simulink model "two_wheel_model_control"  (R2020a)
settings: Solver=VariableStepAuto  StartTime=0.0  StopTime=10.0  RelTol=1e-3
values from neighbouring files (symbols this model uses):
  A23 = -b*d/(a*c-b*e)    (= -1.9886253421)    [two_wheel_model.m]
  A43 = a*d/(a*c-b*e)    (= 33.2052798573)    [two_wheel_model.m]
  B21 = (c+b)/(a*c-b*e)    (= 1.96075852141)    [two_wheel_model.m]
  B22 = (c+b)/(a*c-b*e)    (= 1.96075852141)    [two_wheel_model.m]
  B41 = -(e+a)/(a*c-b*e)    (= -10.2174481788)    [two_wheel_model.m]
  B42 = -(e+a)/(a*c-b*e)    (= -10.2174481788)    [two_wheel_model.m]
  B61 = f    (= 7.73512853901)    [two_wheel_model.m]
  B62 = -f    (= -7.73512853901)    [two_wheel_model.m]
  K = lqr(A,B,Q,R)    [two_wheel_model.m]
  V = 1.5    [two_wheel_model.m]
  Yaw = 0.523    [two_wheel_model.m]
settings Model: Creator=solitude  LastModifiedBy=solitude

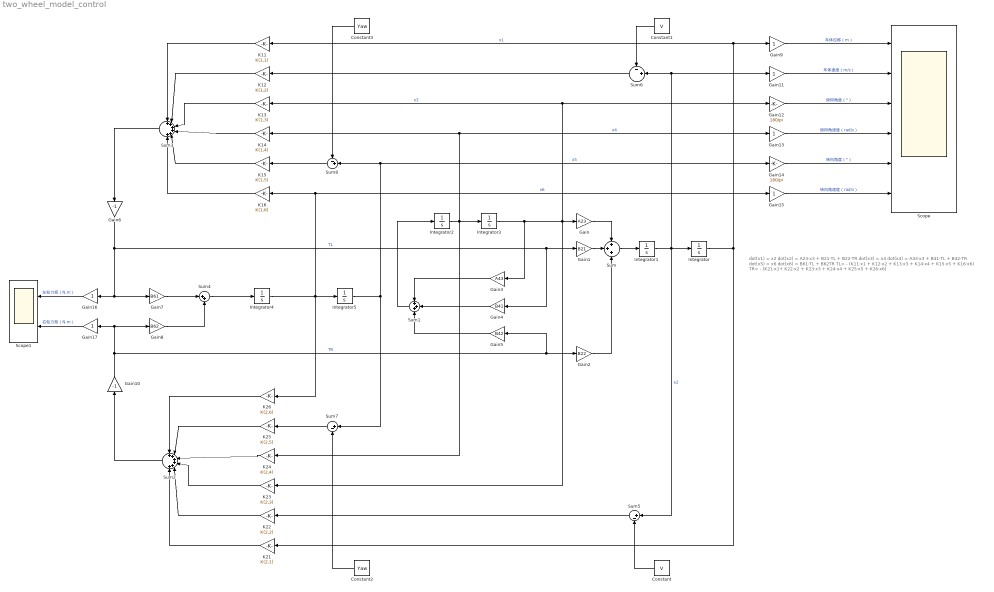
== system two_wheel_model_control ==
  note: dot(x1) = x2
      |
      | dot(x2) = A23·x3 + B21·TL + B22·TR
      |
      | dot(x3) = x4
      |
      | dot(x4) = A43·x3 + B41·TL + B42·TR
      |
      | dot(x5) = x6
      |
      | dot(x6) = B61·TL + B62TR
      |
      | TL= - (K11·x1 + K12·x2 + K13·x3 + K14·x4 + K15·x5 + K16·x6)
      |
      | TR= - (K21·x1+ K22·x2 + K23·x3 + K24·x4 + K25·x5 + K26·x6)
  Constant : Constant  Value=V
  Constant1 : Constant  Value=V
  Constant2 : Constant  Value=Yaw
  Constant3 : Constant  Value=Yaw
  Gain : Gain  Gain=A23
  Gain1 : Gain  Gain=B21
  Gain10 : Gain  Gain=-1
  Gain{9,11,13,15..17} (6 alike) : Gain
  Gain12 : Gain  Gain=180/pi
  Gain14 : Gain  Gain=180/pi
  Gain2 : Gain  Gain=B22
  Gain3 : Gain  Gain=A43
  Gain4 : Gain  Gain=B41
  Gain5 : Gain  Gain=B42
  Gain6 : Gain  Gain=-1
  Gain7 : Gain  Gain=B61
  Gain8 : Gain  Gain=B62
  Integrator{,1..5} (6 alike) : Integrator
  K11 : Gain  Gain=K(1,1)
  K12 : Gain  Gain=K(1,2)
  K13 : Gain  Gain=K(1,3)
  K14 : Gain  Gain=K(1,4)
  K15 : Gain  Gain=K(1,5)
  K16 : Gain  Gain=K(1,6)
  K21 : Gain  Gain=K(2,1)
  K22 : Gain  Gain=K(2,2)
  K23 : Gain  Gain=K(2,3)
  K24 : Gain  Gain=K(2,4)
  K25 : Gain  Gain=K(2,5)
  K26 : Gain  Gain=K(2,6)
  Scope : Scope  NumInputPorts=6
  Scope1 : Scope  NumInputPorts=2
  Sum : Sum  Inputs=+++
  Sum1 : Sum  Inputs=+++
  Sum2 : Sum  Inputs=++++++
  Sum3 : Sum  Inputs=++++++
  Sum4 : Sum  Inputs=|++
  Sum5 : Sum  Inputs=|+-
  Sum6 : Sum  Inputs=-+|
  Sum7 : Sum  Inputs=|+-
  Sum8 : Sum  Inputs=-+|
  wires:
  Integrator/1 -> K11/1, Gain9/1, K21/1  "x1"
  Integrator1/1 -> Sum5/1, Sum6/2, Gain11/1, Integrator/1  "x2"
  Integrator2/1 -> Gain13/1, K14/1, K24/1, Integrator3/1  "x4"
  Integrator3/1 -> Gain3/1, K23/1, Gain12/1, K13/1, Gain/1  "x3"
  Gain/1 -> Sum/1
  Gain1/1 -> Sum/2
  Gain2/1 -> Sum/3
  Gain10/1 -> Gain2/1, Gain5/1, Gain8/1, Gain17/1  "TR"
  Sum/1 -> Integrator1/1
  Gain4/1 -> Sum1/2
  Gain3/1 -> Sum1/1
  Gain5/1 -> Sum1/3
  Sum1/1 -> Integrator2/1
  Sum2/1 -> Gain10/1
  Gain6/1 -> Gain7/1, Gain16/1, Gain4/1, Gain1/1  "TL"
  K11/1 -> Sum3/1
  K12/1 -> Sum3/2
  K13/1 -> Sum3/3
  K14/1 -> Sum3/4
  Sum3/1 -> Gain6/1
  Integrator4/1 -> K26/1, Gain15/1, K16/1, Integrator5/1  "x6"
  Sum4/1 -> Integrator4/1
  Gain7/1 -> Sum4/1
  Gain8/1 -> Sum4/2
  Integrator5/1 -> Sum7/1, Gain14/1, Sum8/2  "x5"
  K15/1 -> Sum3/5
  K16/1 -> Sum3/6
  K21/1 -> Sum2/6
  K22/1 -> Sum2/5
  K23/1 -> Sum2/4
  K24/1 -> Sum2/3
  K25/1 -> Sum2/2
  K26/1 -> Sum2/1
  Sum5/1 -> K22/1
  Constant/1 -> Sum5/2
  Sum6/1 -> K12/1
  Constant1/1 -> Sum6/1
  Sum7/1 -> K25/1
  Constant2/1 -> Sum7/2
  Sum8/1 -> K15/1
  Constant3/1 -> Sum8/1
  Gain9/1 -> Scope/1  "车体位移（m）"
  Gain11/1 -> Scope/2  "车体速度（m/s）"
  Gain12/1 -> Scope/3  "俯仰角度（°）"
  Gain13/1 -> Scope/4  "俯仰角速度（rad/s）"
  Gain14/1 -> Scope/5  "转向角度（°）"
  Gain15/1 -> Scope/6  "转向角速度（rad/s）"
  Gain16/1 -> Scope1/1  "左轮力矩（N.m）"
  Gain17/1 -> Scope1/2  "右轮力矩（N.m）"
